simulink model "mpclinearization"  (Simulink 6.0)
settings: Solver=ode45  StartTime=0.0  StopTime=10.0  RelTol=1e-3
libraries: mpclib x1
settings Model: Creator=jowen  LastModifiedBy=jowen
settings DataIOCC: SignalLoggingName=logsOut
settings DebuggingCC: CheckExecutionContextPreStartOutputMsg=on  CheckExecutionContextRuntimeOutputMsg=on  SolverPrmCheckMsg=none
settings CodeAppCC: MangleLength=5
settings SFSimCC: SFSimApplyToAllLibs=on  SFSimBuildMode=Incremental

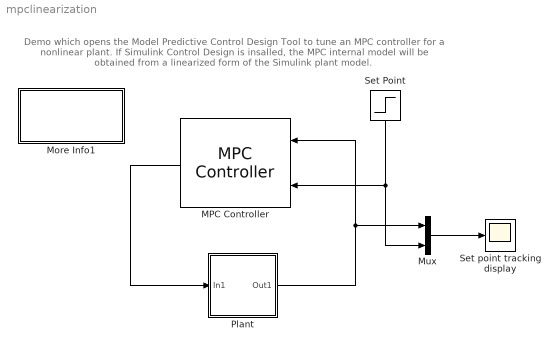
== system mpclinearization ==
  note: Demo which opens the Model Predictive Control Design Tool to tune an MPC controller for a
      | nonlinear plant. If Simulink Control Design is insalled, the MPC internal model will be obtained
      | from a linearized form of the Simulink plant model.
  MPC Controller : mpclib/MPC Controller  Orientation=left  n_mv=1  x0=[]  ref_from_ws=off  ref_signal_name=[]  ref_preview=on  md_from_ws=off  md_signal_name=[]  md_preview=on  from_project=off  md_inport=off  project_file=MPCtask.mat
  More Info1 : Subsystem  PropExecContextAcrossSSBoundary=on
      settings: OpenFcn=mpcdesign_callback('mpclinearization')
      mask Display: disp('Double click\nhere to\nStart')
  Mux : Mux  Inputs=2
  Plant : Subsystem  PropExecContextAcrossSSBoundary=on
  Set Point : Step  Orientation=down  SampleTime=0
  Set point tracking display : Scope
  wires:
  Plant/1(Out1) -> Mux/1, MPC Controller/1
  Set Point/1 -> Mux/2, MPC Controller/2
  Mux/1 -> Set point tracking display/1
  MPC Controller/1 -> Plant/1(In1)

== system mpclinearization/More Info1 ==

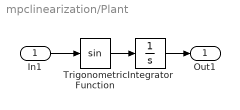
== system mpclinearization/Plant ==
  In1 : Inport  LatchInput=off
  Integrator : Integrator
  Trigonometric Function : Trigonometry
  Out1 : Outport
  wires:
  Trigonometric Function/1 -> Integrator/1
  Integrator/1 -> Out1/1
  In1/1 -> Trigonometric Function/1
